simulink model "PID_test"  (R2022b)
settings: Solver=VariableStepAuto  StartTime=0.0  StopTime=5000  RelTol=1e-3

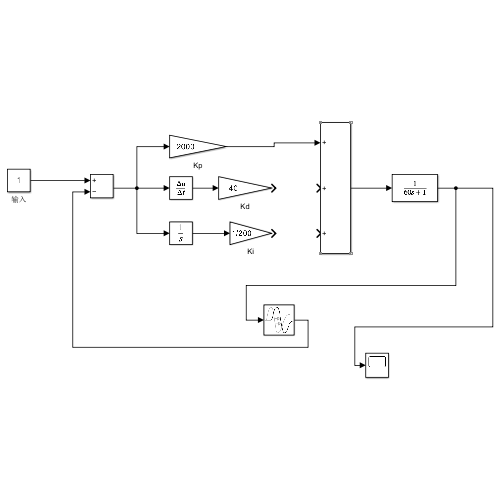
[thumbnail: Simulink's stored preview of the top-level diagram]
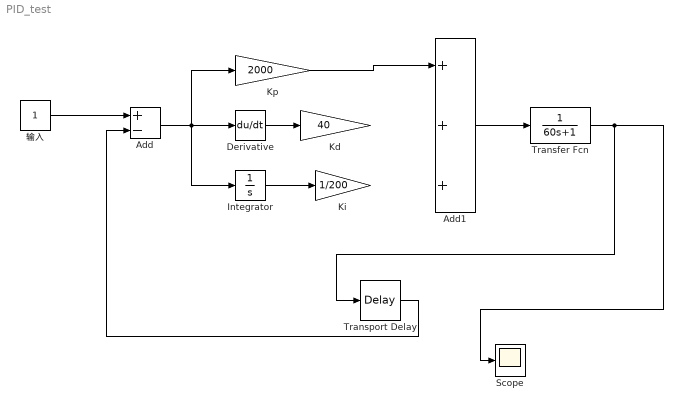
== system PID_test ==
  Add : Sum  Inputs=+-
  Add1 : Sum  Inputs=+++
  Derivative : Derivative
  Integrator : Integrator
  Kd : Gain  Gain=40
  Ki : Gain  Gain=1/200
  Kp : Gain  Gain=2000
  Scope : Scope
  Transfer Fcn : TransferFcn  Denominator=[60 1]
  Transport Delay : TransportDelay  DelayTime=80
  输入 : Constant
  wires:
  输入/1 -> Add/1
  Add/1 -> Integrator/1, Derivative/1, Kp/1
  Derivative/1 -> Kd/1
  Integrator/1 -> Ki/1
  Kp/1 -> Add1/1
  Add1/1 -> Transfer Fcn/1
  Transfer Fcn/1 -> Transport Delay/1, Scope/1
  Transport Delay/1 -> Add/2
